simulink model "SimulLaserDFT"  (R2020a)
settings: Solver=VariableStepAuto  StartTime=0.0  StopTime=Tsim  RelTol=1e-3
values from neighbouring files (symbols this model uses):
  F1 = 85000*2*pi    (= 534070.75111)    [LaserDFT.m]
  F2 = 90000*2*pi    (= 565486.677646)    [LaserDFT.m]
  F3 = 95000*2*pi    (= 596902.604182)    [LaserDFT.m]
  F4 = 100000*2*pi    (= 628318.530718)    [LaserDFT.m]
  F5 = 115000*2*pi    (= 722566.310326)    [LaserDFT.m]
  F6 = 120000*2*pi    (= 753982.236862)    [LaserDFT.m]
  Te = 1/Fe    (= 3.125e-06)    [LaserDFT.m]    (also in ScriptDFT.m = 0.00446428571429)
settings Model: Creator=raveau  LastModifiedBy=raveau

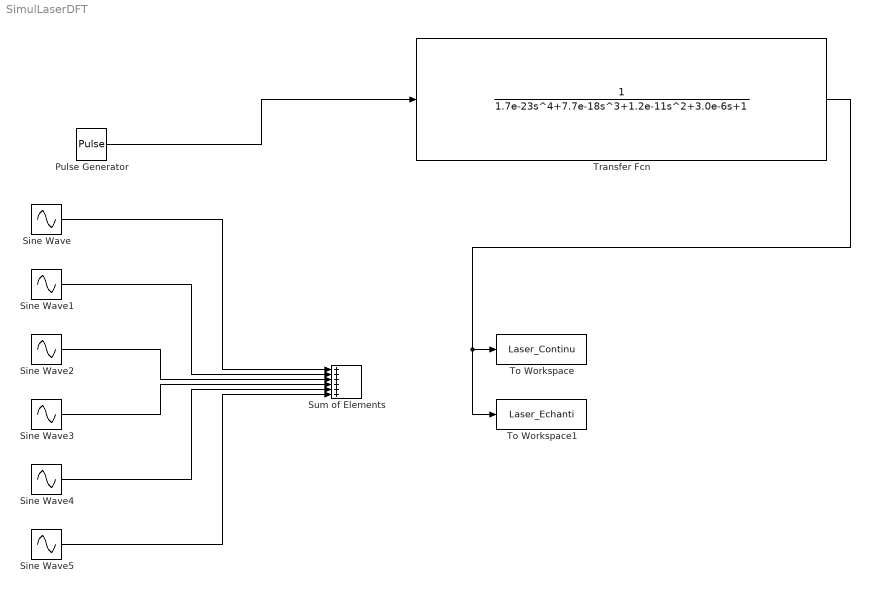
== system SimulLaserDFT ==
  Pulse Generator : DiscretePulseGenerator  PulseType=Time based  Period=1/85000  PulseWidth=50
  Sine Wave : Sin  Frequency=F1  SampleTime=0
  Sine Wave1 : Sin  Frequency=F2  SampleTime=0
  Sine Wave2 : Sin  Frequency=F3  SampleTime=0
  Sine Wave3 : Sin  Frequency=F4  SampleTime=0
  Sine Wave4 : Sin  Frequency=F5  SampleTime=0
  Sine Wave5 : Sin  Frequency=F6  SampleTime=0
  Sum of Elements : Sum  Inputs=++++++
  To Workspace : ToWorkspace  VariableName=Laser_Continu  SaveFormat=Timeseries  SampleTime=Te/100
  To Workspace1 : ToWorkspace  VariableName=Laser_Echanti  SaveFormat=Timeseries  SampleTime=Te
  Transfer Fcn : TransferFcn  Denominator=[1.7e-23 7.7e-18 1.2e-11 3.0e-6 1]
  wires:
  Sine Wave5/1 -> Sum of Elements/6
  Sine Wave4/1 -> Sum of Elements/5
  Sine Wave3/1 -> Sum of Elements/4
  Sine Wave2/1 -> Sum of Elements/3
  Sine Wave1/1 -> Sum of Elements/2
  Sine Wave/1 -> Sum of Elements/1
  Pulse Generator/1 -> Transfer Fcn/1
  Transfer Fcn/1 -> To Workspace1/1, To Workspace/1
